simulink model "vrcmspex"  (Simulink 3.00)
settings: Solver=FixedStepDiscrete  StartTime=0.0  StopTime=10.0  RelTol=1e-3
libraries: smxl x4
settings Model: LastModifiedBy=giampiero

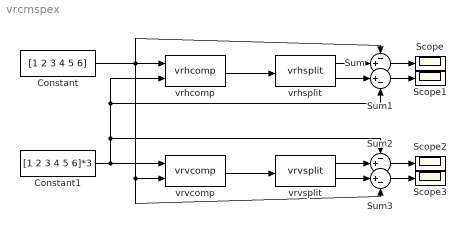
== system vrcmspex ==
  Constant : Constant  Value=[1 2 3 4 5 6]
  Constant1 : Constant  Value=[1 2 3 4 5 6]*3
  Scope{,1..3} (4 alike) : Scope
      Scope settings: TickLabels=off  TimeRange=10  YMin=-1  YMax=1  SaveToWorkspace=off  SaveName=ScopeData
      Scope1 settings: TickLabels=off  TimeRange=10  YMin=-1  YMax=1  SaveToWorkspace=off  SaveName=ScopeData
      Scope2 settings: TickLabels=off  TimeRange=10  YMin=-5e-015  YMax=5e-015  SaveToWorkspace=off  SaveName=ScopeData
      Scope3 settings: TickLabels=off  TimeRange=10  YMin=-5e-015  YMax=5e-015  SaveToWorkspace=off  SaveName=ScopeData
  Sum : Sum  Inputs=-+|  SaturateOnIntegerOverflow=on
  Sum1 : Sum  Inputs=|+-  SaturateOnIntegerOverflow=on
  Sum2 : Sum  Inputs=-+|  SaturateOnIntegerOverflow=on
  Sum3 : Sum  Inputs=|+-  SaturateOnIntegerOverflow=on
  vrhcomp : smxl/Real Matrices/vrhcomp  dims=[3 2 2]
  vrhsplit : smxl/Real Matrices/vrhsplit  dims=[3 2 2]
  vrvcomp : smxl/Real Matrices/vrvcomp  dims=[3 3 2]
  vrvsplit : smxl/Real Matrices/vrvsplit  dims=[3 3 2]
  wires:
  Constant1/1 -> vrvcomp/1, vrhcomp/2, Sum1/2, Sum2/1
  Constant/1 -> vrhcomp/1, Sum/1, vrvcomp/2, Sum3/2
  vrhcomp/1 -> vrhsplit/1
  vrvcomp/1 -> vrvsplit/1
  Sum/1 -> Scope/1
  vrhsplit/1 -> Sum/2
  vrhsplit/2 -> Sum1/1
  Sum1/1 -> Scope1/1
  vrvsplit/1 -> Sum2/2
  vrvsplit/2 -> Sum3/1
  Sum2/1 -> Scope2/1
  Sum3/1 -> Scope3/1
